simulink model "crc_8_optimized_manual"  (R2021b)
settings: Solver=FixedStepDiscrete  StartTime=0.0  StopTime=1  FixedStep=0.01  RelTol=1e-3
libraries: commcrc2 x1
settings Model: Creator=jekyll  LastModifiedBy=jekyll
settings OptimizationCC: DefaultParameterBehavior=Inlined  EnhancedBackFolding=on  PassReuseOutputArgsAs=Individual arguments  OptimizeBlockOrder=speed  DifferentSizesBufferReuse=on  OptimizationCustomize=off  EfficientTunableParamExpr=on
settings DebuggingCC: ParameterTunabilityLossMsg=error
settings SFSimCC: MATLABDynamicMemAlloc=off
settings RTWCC: Description=Embedded Coder  SystemTargetFile=ert.tlc  GenCodeOnly=on  TemplateMakefile=ert_default_tmf
settings CodeAppCC: ForceParamTrailComments=on  IgnoreCustomStorageClasses=off  OperatorAnnotations=on  SimulinkDataObjDesc=on  SFDataObjDesc=on  InsertBlockDesc=on
settings ERTTargetCC: TargetLangStandard=C99 (ISO)  GenerateSampleERTMain=on  SupportAbsoluteTime=off  CodeInterfacePackaging=Reusable function  SupportNonFinite=off  SupportComplex=off  InlinedParameterPlacement=NonHierarchical  ERTCustomFileTemplate=example_file_process.tlc

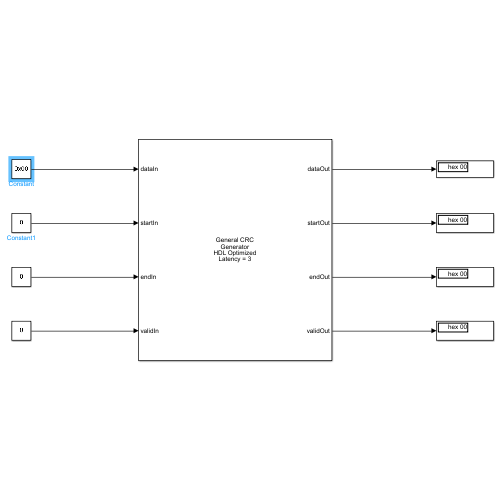
[thumbnail: Simulink's stored preview of the top-level diagram]
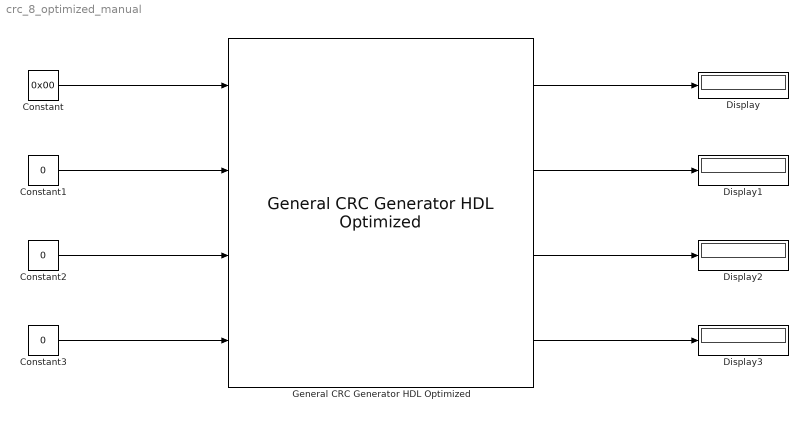
== system crc_8_optimized_manual ==
  Constant : Constant  Value=0x00  OutDataTypeStr=uint8
  Constant1 : Constant  Value=0  OutDataTypeStr=boolean
  Constant2 : Constant  Value=0  OutDataTypeStr=boolean
  Constant3 : Constant  Value=0  OutDataTypeStr=boolean
  Display{,1..3} (4 alike) : Display
      settings: Format=hex (Stored Integer)
  General CRC Generator HDL Optimized : commcrc2/General CRC Generator HDL Optimized  Polynomial=[1, 0, 0, 0, 1, 1, 1 , 0, 1]  InitialState=1  DirectMethod=on  ReflectInput=off  ReflectCRCChecksum=off  FinalXORValue=1  SimulateUsing=Code generation
      settings: SourceProductBaseCode=CM
  wires:
  Constant2/1 -> General CRC Generator HDL Optimized/3
  General CRC Generator HDL Optimized/2 -> Display1/1
  Constant3/1 -> General CRC Generator HDL Optimized/4
  General CRC Generator HDL Optimized/3 -> Display2/1
  Constant/1 -> General CRC Generator HDL Optimized/1
  Constant1/1 -> General CRC Generator HDL Optimized/2
  General CRC Generator HDL Optimized/4 -> Display3/1
  General CRC Generator HDL Optimized/1 -> Display/1
